simulink model "Shagai_Throwing"  (R2019b)
settings: Solver=FixedStepAuto  StartTime=0.0  StopTime=2  FixedStep=0.0005  RelTol=1e-3
values from neighbouring files (symbols this model uses):
  contact_damping = 70    [Shagai_Values.m]
  contact_damping_wood = 400    [Shagai_Values.m]
  contact_stiffness = 500    [Shagai_Values.m]
  contact_stiffness_wood = 10000    [Shagai_Values.m]
  height_mm = 155    [Shagai_Values.m]
  k_fric_plane = 0.6    [Shagai_Values.m]
  k_fric_throw = 0.34    [Shagai_Values.m]
  piston_force = 32    [Shagai_Values.m]
  plane_x = 10    [Shagai_Values.m]
  plane_y = 10    [Shagai_Values.m]
  project_len = 0.55    [Shagai_Values.m]
  s_fric_plane = 0.6    [Shagai_Values.m]
  s_fric_throw = 0.344    [Shagai_Values.m]
  shagai_mass = shagai_mass+50    (= 710)    [Shagai_Values.m]
  theta = theta+0.5    (= 11.5)    [Shagai_Values.m]
  thrower_p_x = 1.06    [Shagai_Values.m]
  thrower_p_y = 0.5    [Shagai_Values.m]
  thrower_x = 0.11    [Shagai_Values.m]
  thrower_y = 0.075    [Shagai_Values.m]
undefined symbols (not defined in the file or in its folder): sigbuilder_block, X, Y, Z
libraries: sm_lib x127, Contact_Forces_Lib x76, nesl_utility x11
(part 6 of 6)

== system Shagai_Throwing/Shagai_Plane_ContactSubsystem/Subsystem4/Face to Plane Force5 ==
  Bus Creator : BusCreator  Inputs=4
  Sphere to Plane Force nz{2..3,6..7} (4 alike) : Contact_Forces_Lib/3D/Sphere to Plane Force  sphere_rad=FacF_rSph  plane_lenx=PlaB_x  plane_leny=PlaB_y  plane_depth=PlaB_z  force_law=Nonlinear  k_contact=k_contact_pla2pla  b_contact=b_contact_pla2pla  pen_full_damp_F=pen_full_damp_F_pla2pla  pen_exponent=pen_exponent_pla2pla  custom_param_1=1  custom_param_2=1  friction_law=Stick-Slip Continuous  mu_kinetic=mu_kinetic_pla2pla  mu_static=mu_static_pla2pla  v_thr=v_thr_pla2pla  vis_on=off  vis_opc_en=0  vis_len_plaBz=vis_len_plaLz  vis_clr=vis_clr  vis_opc=vis_opc
  Transform Fnz10 : sm_lib/Frames and Transforms/Rigid Transform  TranslationMethod=None  TranslationStandardOffset=0  TranslationLengthUnit=m  TranslationStandardAxis=-Z  TranslationCartesianOffset=[FacF_x/2 FacF_y/2 -FacF_z]+[-1 -1 1*sign(FacF_z)]*FacF_rSph  TranslationROffset=0  TranslationROffsetUnits=m  TranslationZOffset=0  TranslationZOffsetUnits=m  TranslationThetaOffset=0  TranslationThetaOffsetUnits=deg  RotationMethod=StandardAxis  RotationAngleUnits=deg  RotationStandardAxis=+Z  RotationAngle=45  RotationArbitraryAxis=[0 0 1]  FollAlignAxisA=+X  BaseAlignAxisA=+Y  FollAlignAxisB=+Y  BaseAlignAxisB=+Z  RotationSequenceAxes=FollowerAxes  RotationSequence=XYX  RotationSequenceAngles=[0 0 0]  RotationSequenceAnglesUnits=deg  RotationMatrix=[1 0 0; 0 1 0; 0 0 1]
  Transform Fnz11 : sm_lib/Frames and Transforms/Rigid Transform  TranslationMethod=None  TranslationStandardOffset=0  TranslationLengthUnit=m  TranslationStandardAxis=-Z  TranslationCartesianOffset=[FacF_x/2 FacF_y/2 -FacF_z]+[-1 -1 1*sign(FacF_z)]*FacF_rSph  TranslationROffset=0  TranslationROffsetUnits=m  TranslationZOffset=0  TranslationZOffsetUnits=m  TranslationThetaOffset=0  TranslationThetaOffsetUnits=deg  RotationMethod=StandardAxis  RotationAngleUnits=deg  RotationStandardAxis=+Z  RotationAngle=45  RotationArbitraryAxis=[0 0 1]  FollAlignAxisA=+X  BaseAlignAxisA=+Y  FollAlignAxisB=+Y  BaseAlignAxisB=+Z  RotationSequenceAxes=FollowerAxes  RotationSequence=XYX  RotationSequenceAngles=[0 0 0]  RotationSequenceAnglesUnits=deg  RotationMatrix=[1 0 0; 0 1 0; 0 0 1]
  Transform Fnz2 : sm_lib/Frames and Transforms/Rigid Transform  TranslationMethod=Cartesian  TranslationStandardOffset=0  TranslationLengthUnit=m  TranslationStandardAxis=-Z  TranslationCartesianOffset=[FacF_x/2 -FacF_y/2 -FacF_z]+[-1 1 1*sign(FacF_z)]*FacF_rSph  TranslationROffset=0  TranslationROffsetUnits=m  TranslationZOffset=0  TranslationZOffsetUnits=m  TranslationThetaOffset=0  TranslationThetaOffsetUnits=deg  RotationMethod=None  RotationAngleUnits=deg  RotationStandardAxis=+Z  RotationAngle=0.0  RotationArbitraryAxis=[0 0 1]  FollAlignAxisA=+X  BaseAlignAxisA=+Y  FollAlignAxisB=+Y  BaseAlignAxisB=+Z  RotationSequenceAxes=FollowerAxes  RotationSequence=XYX  RotationSequenceAngles=[0 0 0]  RotationSequenceAnglesUnits=deg  RotationMatrix=[1 0 0; 0 1 0; 0 0 1]
  Transform Fnz3 : sm_lib/Frames and Transforms/Rigid Transform  TranslationMethod=Cartesian  TranslationStandardOffset=0  TranslationLengthUnit=m  TranslationStandardAxis=-Z  TranslationCartesianOffset=[-FacF_x/2 -FacF_y/2 -FacF_z]+[1 1 1*sign(FacF_z)]*FacF_rSph  TranslationROffset=0  TranslationROffsetUnits=m  TranslationZOffset=0  TranslationZOffsetUnits=m  TranslationThetaOffset=0  TranslationThetaOffsetUnits=deg  RotationMethod=None  RotationAngleUnits=deg  RotationStandardAxis=+Z  RotationAngle=0.0  RotationArbitraryAxis=[0 0 1]  FollAlignAxisA=+X  BaseAlignAxisA=+Y  FollAlignAxisB=+Y  BaseAlignAxisB=+Z  RotationSequenceAxes=FollowerAxes  RotationSequence=XYX  RotationSequenceAngles=[0 0 0]  RotationSequenceAnglesUnits=deg  RotationMatrix=[1 0 0; 0 1 0; 0 0 1]
  Transform Fnz6 : sm_lib/Frames and Transforms/Rigid Transform  TranslationMethod=Cartesian  TranslationStandardOffset=0  TranslationLengthUnit=m  TranslationStandardAxis=-Z  TranslationCartesianOffset=[FacF_x/2 -FacF_y/2 -FacF_z]+[-1 1 1*sign(FacF_z)]*FacF_rSph  TranslationROffset=0  TranslationROffsetUnits=m  TranslationZOffset=0  TranslationZOffsetUnits=m  TranslationThetaOffset=0  TranslationThetaOffsetUnits=deg  RotationMethod=None  RotationAngleUnits=deg  RotationStandardAxis=+Z  RotationAngle=0.0  RotationArbitraryAxis=[0 0 1]  FollAlignAxisA=+X  BaseAlignAxisA=+Y  FollAlignAxisB=+Y  BaseAlignAxisB=+Z  RotationSequenceAxes=FollowerAxes  RotationSequence=XYX  RotationSequenceAngles=[0 0 0]  RotationSequenceAnglesUnits=deg  RotationMatrix=[1 0 0; 0 1 0; 0 0 1]
  Transform Fnz7 : sm_lib/Frames and Transforms/Rigid Transform  TranslationMethod=Cartesian  TranslationStandardOffset=0  TranslationLengthUnit=m  TranslationStandardAxis=-Z  TranslationCartesianOffset=[-FacF_x/2 -FacF_y/2 -FacF_z]+[1 1 1*sign(FacF_z)]*FacF_rSph  TranslationROffset=0  TranslationROffsetUnits=m  TranslationZOffset=0  TranslationZOffsetUnits=m  TranslationThetaOffset=0  TranslationThetaOffsetUnits=deg  RotationMethod=None  RotationAngleUnits=deg  RotationStandardAxis=+Z  RotationAngle=0.0  RotationArbitraryAxis=[0 0 1]  FollAlignAxisA=+X  BaseAlignAxisA=+Y  FollAlignAxisB=+Y  BaseAlignAxisB=+Z  RotationSequenceAxes=FollowerAxes  RotationSequence=XYX  RotationSequenceAngles=[0 0 0]  RotationSequenceAnglesUnits=deg  RotationMatrix=[1 0 0; 0 1 0; 0 0 1]
  PlaB : PMIOPort  Side=Right
  FacF : PMIOPort  Port=2  Side=Left
  Out : Outport  VectorParamsAs1DForOutWhenUnconnected=off
  wires:
  Sphere to Plane Force nz7/1 -> Bus Creator/4  "fz5"
  Sphere to Plane Force nz6/1 -> Bus Creator/3  "fz4"
  Sphere to Plane Force nz2/1 -> Bus Creator/1  "fz2"
  Sphere to Plane Force nz3/1 -> Bus Creator/2  "fz3"
  Bus Creator/1 -> Out/1
  connections:
  Transform Fnz6/LConn1 -- Transform Fnz10/RConn1
  Transform Fnz10/LConn1 -- FacF/RConn1 -- Transform Fnz11/LConn1 -- Transform Fnz3/LConn1 -- Transform Fnz2/LConn1
  Transform Fnz7/LConn1 -- Transform Fnz11/RConn1
  Sphere to Plane Force nz7/LConn1 -- Transform Fnz7/RConn1
  Sphere to Plane Force nz6/LConn1 -- Transform Fnz6/RConn1
  Sphere to Plane Force nz7/RConn1 -- Sphere to Plane Force nz6/RConn1 -- Sphere to Plane Force nz2/RConn1 -- Sphere to Plane Force nz3/RConn1 -- PlaB/RConn1
  Sphere to Plane Force nz2/LConn1 -- Transform Fnz2/RConn1
  Sphere to Plane Force nz3/LConn1 -- Transform Fnz3/RConn1
